simulink model "model_1"  (R2018b)
settings: Solver=VariableStepAuto  StartTime=0.0  StopTime=10.0  RelTol=1e-3
undefined symbols (not defined in the file or in its folder): A, C
settings Model: Creator=mariu  LastModifiedBy=mariu

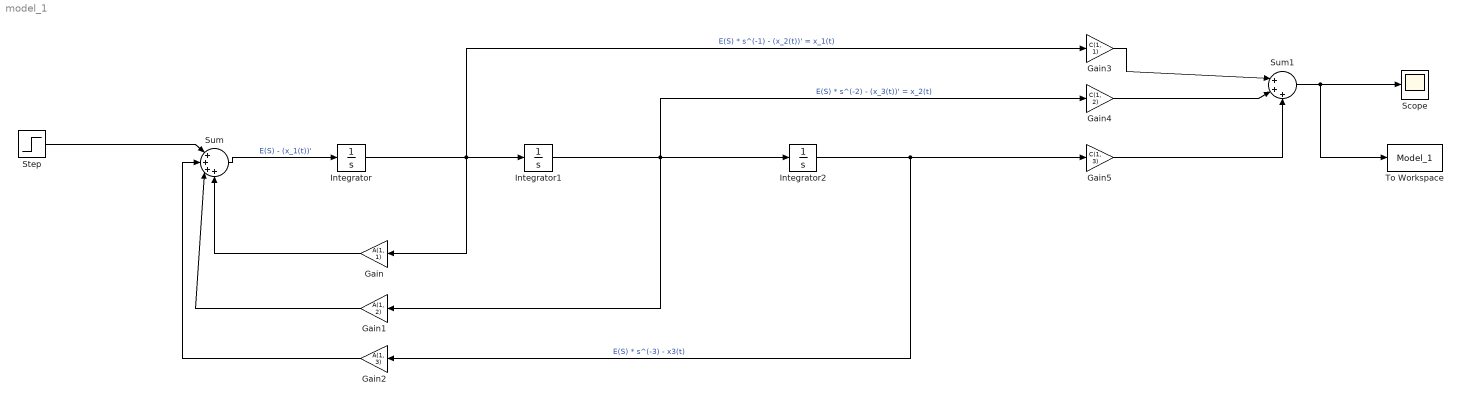
== system model_1 ==
  Gain : Gain  Gain=A(1, 1)
  Gain1 : Gain  Gain=A(1, 2)
  Gain2 : Gain  Gain=A(1, 3)
  Gain3 : Gain  Gain=C(1, 1)
  Gain4 : Gain  Gain=C(1, 2)
  Gain5 : Gain  Gain=C(1, 3)
  Integrator : Integrator
  Integrator1 : Integrator
  Integrator2 : Integrator
  Scope : Scope
  Step : Step  SampleTime=0
  Sum : Sum  Inputs=|++++
      settings: AttributesFormatString=%<Inputs>
  Sum1 : Sum  Inputs=|+++
      settings: AttributesFormatString=%<Inputs>
  To Workspace : ToWorkspace  VariableName=Model_1  SaveFormat=Timeseries  SampleTime=-1
  wires:
  Sum/1 -> Integrator/1  "E(S) - (x_1(t))'"
  Integrator/1 -> Gain3/1, Gain/1, Integrator1/1  "E(S) * s^(-1) - (x_2(t))' = x_1(t)"
  Integrator1/1 -> Gain4/1, Gain1/1, Integrator2/1  "E(S) * s^(-2) - (x_3(t))' = x_2(t)"
  Integrator2/1 -> Gain5/1, Gain2/1  "E(S) * s^(-3) - x3(t)"
  Gain2/1 -> Sum/2
  Gain/1 -> Sum/4
  Gain1/1 -> Sum/3
  Step/1 -> Sum/1
  Gain3/1 -> Sum1/1
  Gain4/1 -> Sum1/2
  Gain5/1 -> Sum1/3
  Sum1/1 -> To Workspace/1, Scope/1
